simulink model "modell"  (Simulink 7.3)
settings: Solver=ode4  StartTime=0.0  StopTime=Inf  RelTol=1e-3
values from neighbouring files (symbols this model uses):
  A_w = [zeros(3) eye(3) ... (first row only)    [data.m]
  C_w = [zeros(3) eye(3)]    [data.m]
  D_i = 1*[2    0       0 ... (first row only)    [data.m]
  E_b_i = diag([1 1 1])    [data.m]
  E_b_s = diag([1 1 1])    [data.m]
  K_1 = debug*[diag([-2.2   -2.2    -2.2]) ... (first row only)    [data.m]
  K_2 = debug*0.001*diag([1 1 1])    [data.m]
  K_3 = debug*0.001*diag([0.01 0.01 0.001])    [data.m]
  K_4 = debug*0.001*diag([0.1 0.1 0.1])    [data.m]
  Ke = 100*diag([1.28 1.05 1.28 1.05 2.14])    [data.m]    (also in parameeters.m = diag([1.28 1.05 1.28 1.05 2.14]))
  M_i = 1*[25.8     0       0 ... (first row only)    [data.m]
  pos_0_i = [0, 0, 0]'    [data.m]
  pos_diff = pos_0_s - pos_0_i    [data.m]
  T_i = diag([1000, 1000, 1000])    [data.m]
  T_s = diag([1000, 1000, 1000])    [data.m]
  T_s_inv = T_s^(-1)    [data.m]
  Te = [1     0       1       0       0 ... (first row only)    [data.m]    (also in parameeters.m = [1 0 1 0 0; 0 1 0 1 1; ly1 -lx1 -ly2 -lx2 lx3])
undefined symbols (not defined in the file or in its folder): D, M
libraries: marine_gnc x13, simulink x5, simulink_extras x2
(part 2 of 2)

== system modell/PS3 Sixaxis/threshold block2/else ==
  In1 : Inport  OutDataType=fixdt(1, 16)  OutScaling=2^0
  Action Port : ActionPort  ActionType=else
  Out1 : Outport  OutDataType=fixdt(1, 16)  OutScaling=2^0
  wires:
  In1/1 -> Out1/1

== system modell/PS3 Sixaxis/threshold block2/if ==
  In1 : Inport  OutDataType=fixdt(1, 16)  OutScaling=2^0
  Action Port : ActionPort  ActionType=then
  Out1 : Outport  OutDataType=fixdt(1, 16)  OutScaling=2^0
  wires:
  In1/1 -> Out1/1

== system modell/PS3 Sixaxis/threshold block3/else ==
  In1 : Inport  OutDataType=fixdt(1, 16)  OutScaling=2^0
  Action Port : ActionPort  ActionType=else
  Out1 : Outport  OutDataType=fixdt(1, 16)  OutScaling=2^0
  wires:
  In1/1 -> Out1/1

== system modell/PS3 Sixaxis/threshold block3/if ==
  In1 : Inport  OutDataType=fixdt(1, 16)  OutScaling=2^0
  Action Port : ActionPort  ActionType=then
  Out1 : Outport  OutDataType=fixdt(1, 16)  OutScaling=2^0
  wires:
  In1/1 -> Out1/1

== system modell/Towline/Towline dynamics/cartesian length ==
  In1 : Inport  OutDataType=fixdt(1, 16)  OutScaling=2^0
  Demux : Demux  Outputs=3
  Sum : Sum  OutDataType=fixdt(1, 16)  OutScaling=2^0
  mf1 : Math  Operator=square  OutDataType=fixdt(1, 16)  OutScaling=2^0  SaturateOnIntegerOverflow=on
  mf2 : Math  Operator=square  OutDataType=fixdt(1, 16)  OutScaling=2^0  SaturateOnIntegerOverflow=on
  mf3 : Math  Operator=sqrt  OutDataType=fixdt(1, 16)  OutScaling=2^0  SaturateOnIntegerOverflow=on
  Out1 : Outport  OutDataType=fixdt(1, 16)  OutScaling=2^0
  wires:
  In1/1 -> Demux/1
  Demux/1 -> mf1/1
  Demux/2 -> mf2/1
  mf2/1 -> Sum/2
  mf1/1 -> Sum/1
  Sum/1 -> mf3/1
  mf3/1 -> Out1/1

== system modell/Towline/Towline dynamics/cartesian length1 ==
  In1 : Inport  OutDataType=fixdt(1, 16)  OutScaling=2^0
  Demux : Demux  Outputs=3
  Sum : Sum  OutDataType=fixdt(1, 16)  OutScaling=2^0
  mf1 : Math  Operator=square  OutDataType=fixdt(1, 16)  OutScaling=2^0  SaturateOnIntegerOverflow=on
  mf2 : Math  Operator=square  OutDataType=fixdt(1, 16)  OutScaling=2^0  SaturateOnIntegerOverflow=on
  mf3 : Math  Operator=sqrt  OutDataType=fixdt(1, 16)  OutScaling=2^0  SaturateOnIntegerOverflow=on
  Out1 : Outport  OutDataType=fixdt(1, 16)  OutScaling=2^0
  wires:
  In1/1 -> Demux/1
  Demux/1 -> mf1/1
  Demux/2 -> mf2/1
  mf2/1 -> Sum/2
  mf1/1 -> Sum/1
  Sum/1 -> mf3/1
  mf3/1 -> Out1/1

== system modell/Towline/Towline dynamics/rupture ==
  In1 : Inport  OutDataType=fixdt(1, 16)  OutScaling=2^0
  Action Port : ActionPort  ActionType=elseif
  Out1 : Outport  OutDataType=fixdt(1, 16)  OutScaling=2^0
  wires:
  In1/1 -> Out1/1

== system modell/Towline/Towline dynamics/slack ==
  In1 : Inport  OutDataType=fixdt(1, 16)  OutScaling=2^0
  Action Port : ActionPort  ActionType=then
  Out1 : Outport  OutDataType=fixdt(1, 16)  OutScaling=2^0
  wires:
  In1/1 -> Out1/1

== system modell/Towline/Towline dynamics/towing ==
  In1 : Inport  OutDataType=fixdt(1, 16)  OutScaling=2^0
  Action Port : ActionPort  ActionType=else
  Out1 : Outport  OutDataType=fixdt(1, 16)  OutScaling=2^0
  wires:
  In1/1 -> Out1/1
